simulink model "CesiumTest"  (R2024b)
settings: Solver=VariableStepAuto  StartTime=0.0  StopTime=inf  RelTol=1e-3
libraries: aerolibsim3d x2, sim3dlib x1
settings Model: Creator=frostydev  LastModifiedBy=frostydev

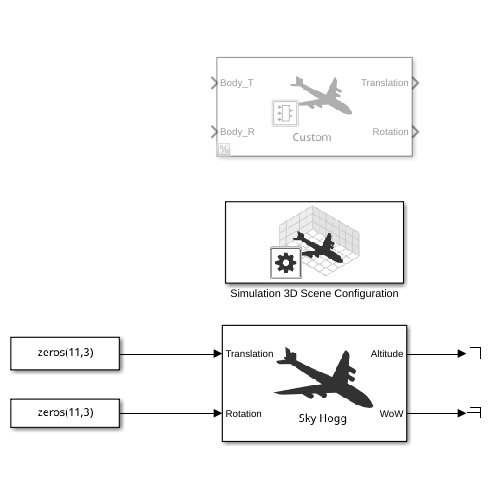
[thumbnail: Simulink's stored preview of the top-level diagram]
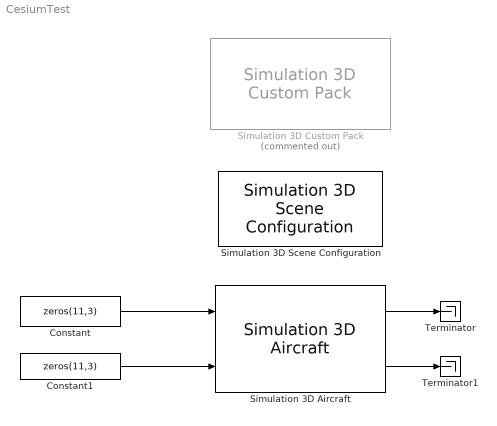
== system CesiumTest ==
  Constant : Constant  Value=zeros(11,3)
  Constant1 : Constant  Value=zeros(11,3)
  Simulation 3D Aircraft : aerolibsim3d/Simulation 3D Aircraft  Priority=-1  Mesh=Sky Hogg  MeshPath=/MathWorksAerospaceContent/Vehicles/Aircraft/Custom/Mesh/SK_HL20.SK_HL20  MeshPathAT=/MathWorksAerospaceContent/Vehicles/Aircraft/AirTransport/Mesh/SK_AirTransport.SK_AirTransport  MeshPathGA=/MathWorksAerospaceContent/Vehicles/Aircraft/GeneralAviation/Mesh/SK_GeneralAviation.SK_GeneralAviation  AircraftColor=Green  ActorName=SimulinkVehicle1  Translation=zeros( 11, 3 )  Rotation=zeros( 11, 3 )  ScaleInputPort=Dialog  Scale=[1 1 1]  InitialScale=[1 1 1]  IsGHSensorEnabled=on  AreGHRaysVisible=off  IsOutputReshapeEnabled=off  GHRayLength=1524  GHBodyOffset=0.90  GHFrontTireRadius=0.21  GHLeftTireRadius=0.21  GHRightTireRadius=0.21  WoWSensorTolerance=0.05  LightsConfig=Automatic lights  LandingLightIntensity=300000  LandingLightConeAngle=15  CustomLeftLandingLightLocation=[0 0 0]  CustomLeftLandingLightOrientation=[0 0 0]  CustomRightLandingLightLocation=[0 0 0]  CustomRightLandingLightOrientation=[0 0 0]  TaxiLightIntensity=150000  TaxiLightConeAngle=36  CustomTaxiLightLocation=[0 0 0]  CustomTaxiLightOrientation=[0 0 0]  NavLightIntensity=500  PositionLightIntensity=500  StrobeLightIntensity=5000  WingtipStrobePeriod=1.5  WingtipStrobePulseWidth=6  TailStrobePeriod=1.5  TailStrobePulseWidth=6  BeaconLightIntensity=4000  BeaconPeriod=1.5  BeaconPulseWidth=10  SampleTime=-1  ActorType=SimulinkVehicle  ID=1  aMode=0  ActorTag=SimulinkVehicle1
  Simulation 3D Custom Pack : aerolibsim3d/Simulation 3D Custom Pack  Commented=on  Engine1_T=off  Engine1_R=off  Engine1_Prop_T=off  Engine1_Prop_R=off  Engine2_T=off  Engine2_R=off  Engine2_Prop_T=off  Engine2_Prop_R=off  Engine3_T=off  Engine3_R=off  Engine3_Prop_T=off  Engine3_Prop_R=off  Engine4_T=off  Engine4_R=off  Engine4_Prop_T=off  Engine4_Prop_R=off  Engine5_T=off  Engine5_R=off  Engine5_Prop_T=off  Engine5_Prop_R=off  Engine6_T=off  Engine6_R=off  Engine6_Prop_T=off  Engine6_Prop_R=off  Engine7_T=off  Engine7_R=off  Engine7_Prop_T=off  Engine7_Prop_R=off  Engine8_T=off  Engine8_R=off  Engine8_Prop_T=off  Engine8_Prop_R=off  Engine9_T=off  Engine9_R=off  Engine9_Prop_T=off  Engine9_Prop_R=off  Engine10_T=off  Engine10_R=off  Engine10_Prop_T=off  Engine10_Prop_R=off  Engine11_T=off  Engine11_R=off  Engine11_Prop_T=off  Engine11_Prop_R=off  Engine12_T=off  Engine12_R=off  Engine12_Prop_T=off  Engine12_Prop_R=off  Engine13_T=off  Engine13_R=off  Engine13_Prop_T=off  Engine13_Prop_R=off  Engine14_T=off  Engine14_R=off  Engine14_Prop_T=off  Engine14_Prop_R=off  Engine15_T=off  Engine15_R=off  Engine15_Prop_T=off  Engine15_Prop_R=off  Engine16_T=off  Engine16_R=off  Engine16_Prop_T=off  Engine16_Prop_R=off  Wing1_T=off  Wing1_R=off  Wing1_Left_Flap_T=off  Wing1_Left_Flap_R=off  Wing1_Right_Flap_T=off  Wing1_Right_Flap_R=off  Wing1_Left_Aileron_T=off  Wing1_Left_Aileron_R=off  Wing1_Right_Aileron_T=off  Wing1_Right_Aileron_R=off  Wing1_Left_Spoiler_T=off  Wing1_Left_Spoiler_R=off  Wing1_Right_Spoiler_T=off  Wing1_Right_Spoiler_R=off  Wing2_T=off  Wing2_R=off  Wing2_Left_Flap_T=off  Wing2_Left_Flap_R=off  Wing2_Right_Flap_T=off  Wing2_Right_Flap_R=off  Horizontal_Stab_T=off  Horizontal_Stab_R=off  Left_Elevator_T=off  Left_Elevator_R=off  Right_Elevator_T=off  Right_Elevator_R=off  Left_Rudder_T=off  Left_Rudder_R=off  Right_Rudder_T=off  Right_Rudder_R=off  Nose_Gear_T=off  Nose_Gear_R=off  Nose_Wheel_T=off  Nose_Wheel_R=off  Nose_Gear_Door_T=off  Nose_Gear_Door_R=off  Left_Gear_T=off  Left_Gear_R=off  Left_Wheel_T=off  Left_Wheel_R=off  Left_Gear_Door_T=off  Left_Gear_Door_R=off  Right_Gear_T=off  Right_Gear_R=off  Right_Wheel_T=off  Right_Wheel_R=off  Right_Gear_Door_T=off  Right_Gear_Door_R=off  GeoRadioButton=NED  AdjustForCesium=off  Heading0=90
  Simulation 3D Scene Configuration : sim3dlib/Simulation 3D Scene Configuration  Priority=0  ProjectFormat=Default Scenes  SceneDesc=Geospatial  ProjectName=/usr/local/MATLAB/R2024b/toolbox/shared/sim3d_projects/automotive_project_linux/UE/LinuxNoEditor/VehicleSimulation.sh  ScenePath=/Game/Maps/HwStrght  EnableOpenDRIVE=off  vehTagList={'Custom';'Scene Origin';'SimulinkVehicle1'}  vehTag=SimulinkVehicle1  FreeCameraInitialTranslation=[-6, 0, 2]  FreeCameraDefaultInitialTranslation=[-6, 0, 2]  FreeCameraInitialRotation=[0, -15, 0]  FreeCameraDefaultInitialRotation=[0, -15, 0]  OpVisEn=off  Ts=.02  EnableWindow=on  EnableRemoteAccess=off  EnableWeather=off  SunAzimuth=90  SunAltitude=40.0  EnableGeospatialSun=off  Latitude=0  Longitude=0  Date=2023-01-01  Time=10:30:00  GeoTimeZone=-5.0  SunDaylightSaving=off  wind=1  clouds=10  EnableVolumetricClouds=off  CloudCoverage=0  CloudAltitude=6  fog=0  rain=0  RaindropsEffect=off  SnowDensity=0  EnableGeospatial=on  AccessTokenID=MatlabSim  UseTrueOrigin=off  OriginHeight=3000  OriginLatitude=41.892469  OriginLongitude=-87.643373  MapStyle=Aerial  AdditionalAssetIDs=[96188]  UseAdvancedSunSky=on  SolarTime=8.25  TimeZone=-5  Day=21  Month=9  Year=2022  UseDaylightSavingTime=on  DSTStartDay=10  DSTStartMonth=3  DSTEndDay=3  DSTEndMonth=11  DSTSwitchHour=2  sensorTag=MainCamera1  sensorId=1  sensorName=MainCamera1  mountLoc=Origin  offsetFlag=off  tmountOffset=[0, 0, 0]  rmountOffset=[0, 0, 0]  HorizontalResolution=1280  VerticalResolution=720  HorizontalFOV=60  mountPoint=[0 0 0]  mountOrientation=[0 0 0]  aMode=0  ID=1  GeoTrigger=Inactive
      settings: LibrarySourceBlock=aerolibsim3d/Simulation 3D Scene Configuration
  Terminator : Terminator
  Terminator1 : Terminator
  wires:
  Simulation 3D Aircraft/1 -> Terminator/1
  Simulation 3D Aircraft/2 -> Terminator1/1
  Constant/1 -> Simulation 3D Aircraft/1
  Constant1/1 -> Simulation 3D Aircraft/2
